simulink model "ch2ex5"  (Simulink 10.2)
settings: Solver=ode15s  StartTime=0.0  StopTime=10  RelTol=1e-3
model workspace (MAT data in the model file):
  Ks = Simulink.Parameter
  Ks.Value = 10000
  Ks.DataType = 'auto'
  Ks.DocUnits = 'N/m'
  Ks.Dimensions = [1 1]
  Kw = Simulink.Parameter
  Kw.Value = 500000
  Kw.DataType = 'auto'
  Kw.DocUnits = 'N/m'
  Kw.Dimensions = [1 1]
  M1 = Simulink.Parameter
  M1.Value = 10
  M1.DataType = 'auto'
  M1.DocUnits = 'kg'
  M1.Dimensions = [1 1]
  M2 = Simulink.Parameter
  M2.Value = 250
  M2.DataType = 'auto'
  M2.DocUnits = 'kg'
  M2.Dimensions = [1 1]
  b = Simulink.Parameter
  b.Value = 1000
  b.DataType = 'auto'
  b.Dimensions = [1 1]
libraries: simulink x1
settings Model: Creator=Tobias  LastModifiedBy=Tobias  OrderedModelArguments=off
settings DataIOCC: SaveFormat=Dataset  SignalLoggingSaveFormat=Dataset  ReturnWorkspaceOutputs=on
settings OptimizationCC: LifeSpan=auto
settings DebuggingCC: UnderspecifiedInitializationDetection=Simplified  MergeDetectMultiDrivingBlocksExec=error  FcnCallInpInsideContextMsg=error  SFUnexpectedBacktrackingDiag=error  SFNoUnconditionalDefaultTransitionDiag=error  SFExecutionAtInitializationDiag=warning  ArithmeticOperatorsInVariantConditions=error
settings HardwareCC: ProdBitPerPointer=64  ProdBitPerSizeT=64  ProdBitPerPtrDiffT=64  ProdLargestAtomicFloat=Float  ProdIntDivRoundTo=Zero  ProdEndianess=LittleEndian  ProdWordSize=64  ProdHWDeviceType=Intel->x86-64 (Windows64)
settings ModelReferenceCC: PropagateSignalLabelsOutOfModel=on
settings SFSimCC: SimUseLocalCustomCode=on  CustomCodeUndefinedFunction=FilterOut
settings RTWCC: RTWUseLocalCustomCode=on
settings CodeAppCC: StateflowObjectComments=off
settings GRTTargetCC: TargetLangStandard=C99 (ISO)  CombineOutputUpdateFcns=on  GRTInterface=off
settings ConfigComp: CovMetricSettings=dwe  CovSaveCumulativeToWorkspaceVar=off  CovSaveSingleToWorkspaceVar=off  CovExternalEMLEnable=on

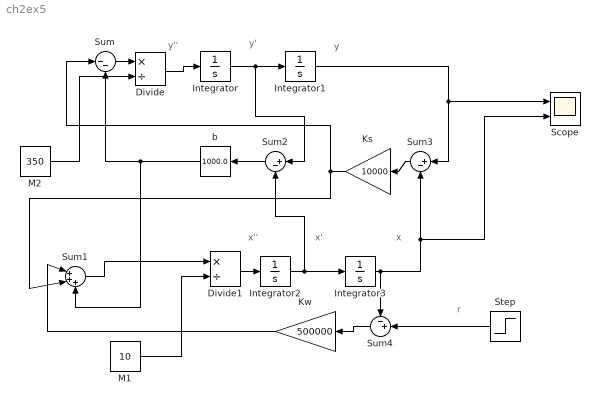
== system ch2ex5 ==
  note: r
  note: x
  note: x'
  note: x''
  note: y
  note: y'
  note: y''
  Divide : Product  Inputs=*/
  Divide1 : Product  Inputs=*/
  Integrator{,1..3} (4 alike) : Integrator
  Ks : Gain  Gain=10000
  Kw : Gain  Gain=500000
  M1 : Constant  Value=10  SampleTime=10
  M2 : Constant  Value=350  SampleTime=10000
  Scope : Scope  NumInputPorts=2
  Step : Step  Time=2  After=2  SampleTime=0
  Sum : Sum  Inputs=|--
  Sum1 : Sum  Inputs=|+++
  Sum2 : Sum  Inputs=|+-
  Sum3 : Sum  Inputs=|+-
  Sum4 : Sum  Inputs=-+|
  b : simulink/Math Operations/Slider Gain  gain=1000.0  low=0  high=10000
  wires:
  Integrator/1 -> Sum2/1, Integrator1/1
  Integrator1/1 -> Sum3/1, Scope/1
  Integrator2/1 -> Integrator3/1, Sum2/2
  Integrator3/1 -> Scope/2, Sum3/2, Sum4/1
  Sum2/1 -> b/1
  M2/1 -> Divide/2
  Sum3/1 -> Ks/1
  Divide/1 -> Integrator/1
  Sum/1 -> Divide/1
  Sum4/1 -> Kw/1
  Divide1/1 -> Integrator2/1
  Sum1/1 -> Divide1/1
  Kw/1 -> Sum1/1
  Step/1 -> Sum4/2
  M1/1 -> Divide1/2
  Ks/1 -> Sum/1, Sum1/2
  b/1 -> Sum1/3, Sum/2
